simulink model "SEGWAY_RT_SFR"  (R2015a)
settings: Solver=ode4  SolverMode=SingleTasking  StartTime=0.0  StopTime=inf  FixedStep=ts  RelTol=1e-3
values from neighbouring files (symbols this model uses):
  Kcd = place(Ad, Bd, polosd_lc)    [Control_Segway_2015.m]    (also in ensayo1.mat = [-68.2484140277 -10.6212069049 -81.1609824123]; ensayo2_wn4.8_seta_0.7.mat = [-20.5032172519 -3.21085847646 -25.3008871114]; ensayo3_wn5.3_seta_0.55.mat = [-22.2986458352 -3.45646199395 -23.8255259596]; ensayo3_wn5.5_seta_0.7.mat = [-22.2599657852 -3.62971388524 -28.5561648788])
  R = 81.6e-3/2    (= 0.0408)    [CONTROL_SEGWAY.m]    (also in Control_Segway_2015.m; ensayo1.mat; ensayo2_wn4.8_seta_0.7.mat; ensayo3_wn5.3_seta_0.55.mat)
  sound_freq = 440    [CONTROL_SEGWAY.m]    (also in Control_Segway_2015.m; ensayo1.mat; ensayo2_wn4.8_seta_0.7.mat; ensayo3_wn5.3_seta_0.55.mat)
  time_start = 1    [CONTROL_SEGWAY.m]    (also in Control_Segway_2015.m; ensayo1.mat; ensayo2_wn4.8_seta_0.7.mat; ensayo3_wn5.3_seta_0.55.mat)
  ts = 5e-3    (= 0.005)    [CONTROL_SEGWAY.m]    (also in Control_Segway_2015.m; ensayo1.mat; ensayo2_wn4.8_seta_0.7.mat; ensayo3_wn5.3_seta_0.55.mat)
  W = 0.15    [CONTROL_SEGWAY.m]    (also in Control_Segway_2015.m; ensayo1.mat; ensayo2_wn4.8_seta_0.7.mat; ensayo3_wn5.3_seta_0.55.mat)
undefined symbols (not defined in the file or in its folder): th
undefined symbols (not defined in the file): alfa1, gyro0
libraries: legonxtlib x16, simulink x4
settings Model: SimulationMode=external  CovSFcnEnable=off  ExtModeTrigDuration=2  Creator=jrperez  LastModifiedBy=stic
settings DataIOCC: SignalLoggingSaveFormat=ModelDataLogs
settings OptimizationCC: ExpressionDepthLimit=2147483647  OptimizeModelRefInitCode=on  LifeSpan=1
settings DebuggingCC: UnderspecifiedInitializationDetection=Classic  MergeDetectMultiDrivingBlocksExec=none  ParameterPrecisionLossMsg=none  FcnCallInpInsideContextMsg=EnableAllAsWarning  StateNameClashWarn=warning
settings HardwareCC: ProdLargestAtomicInteger=Long  ProdLargestAtomicFloat=Float  ProdEndianess=LittleEndian  ProdHWDeviceType=ARM Compatible->ARM 7
settings RTWCC: SystemTargetFile=realtime.tlc  GenerateMakefile=off  TemplateMakefile=realtime.tmf  Description=Real-Time Toolbox  RTWVerbose=off
settings CodeAppCC: CustomSymbolStrType=$N$R$M  InternalIdentifier=Classic
settings ERTTargetCC: CombineOutputUpdateFcns=off  ExtMode=on  ExtModeTransport=1  ExtModeMexFile=ext_serial_win32_comm_no_acks_rtt_byteswap  ExtModeMexArgs=0 4 9600  ERTSrcFileBannerTemplate=realtime_code_template.cgt  ERTHdrFileBannerTemplate=realtime_code_template.cgt  ERTDataSrcFileTemplate=realtime_code_template.cgt  ERTDataHdrFileTemplate=realtime_code_template.cgt  ERTCustomFileTemplate=realtime_file_process.tlc

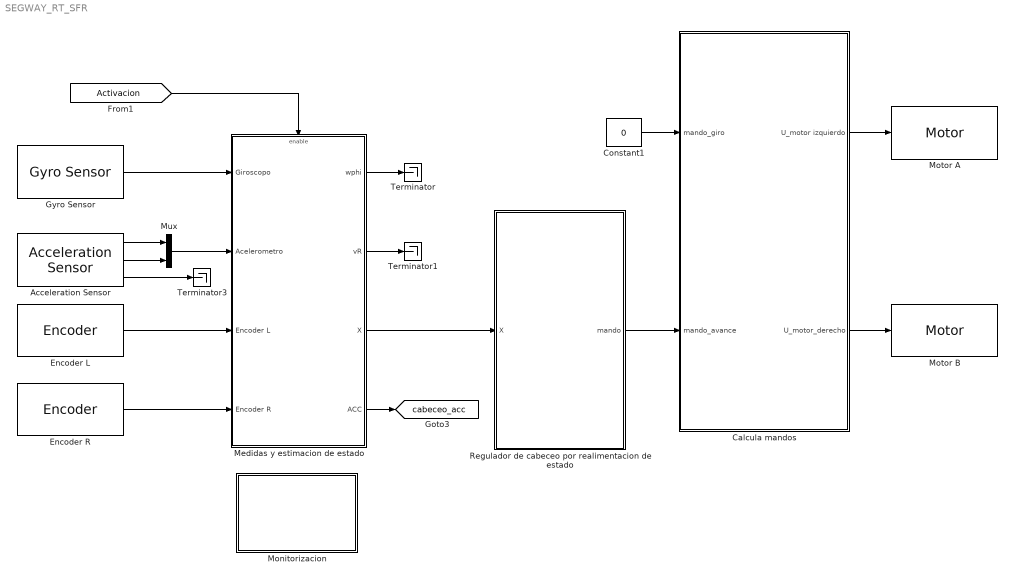
== system SEGWAY_RT_SFR ==
  Acceleration Sensor : legonxtlib/Acceleration Sensor  portNumber=2  sampleTime=ts  blockPlatform=LegoMindstormsNXT
  Calcula mandos : Subsystem
  Constant1 : Constant  Value=0  OutDataTypeStr=single  SampleTime=ts
  Encoder L : legonxtlib/Encoder  portNumber=B  opMode=No reset  sampleTime=ts  blockPlatform=LegoMindstormsNXT
  Encoder R : legonxtlib/Encoder  portNumber=C  opMode=No reset  sampleTime=ts  blockPlatform=LegoMindstormsNXT
  Gyro Sensor : legonxtlib/Gyro Sensor  portNumber=3  outputMode=Raw A/D (0 - 1023)  offset=600  sampleTime=ts  blockPlatform=LegoMindstormsNXT
  Medidas y estimacion de estado : Subsystem
  Monitorizacion : Subsystem
  Motor A : legonxtlib/Motor  sportNumber=B  sstopAction=Brake  blockPlatform=LegoMindstormsNXT
  Motor B : legonxtlib/Motor  sportNumber=C  sstopAction=Brake  blockPlatform=LegoMindstormsNXT
  Mux : Mux  Inputs=2
  Regulador de cabeceo por realimentacion de estado : Subsystem
  Terminator : Terminator
  Terminator1 : Terminator
  Terminator3 : Terminator
  tag scope: cabeceo_acc=global
  wires:
  Gyro Sensor/1 -> Medidas y estimacion de estado/1(Giroscopo)
  Encoder L/1 -> Medidas y estimacion de estado/3(Encoder L)
  Calcula mandos/1(U_motor izquierdo) -> Motor A/1
  Calcula mandos/2(U_motor_derecho) -> Motor B/1
  Encoder R/1 -> Medidas y estimacion de estado/4(Encoder R)
  Medidas y estimacion de estado/3(X) -> Regulador de cabeceo por realimentacion de estado/1(X)
  [Activacion] -> Medidas y estimacion de estado/Enable
  Constant1/1 -> Calcula mandos/1(mando_giro)
  Regulador de cabeceo por realimentacion de estado/1(mando) -> Calcula mandos/2(mando_avance)
  Medidas y estimacion de estado/1(wphi) -> Terminator/1
  Medidas y estimacion de estado/2(vR) -> Terminator1/1
  Acceleration Sensor/3 -> Terminator3/1
  Medidas y estimacion de estado/4(ACC) -> [cabeceo_acc]
  Acceleration Sensor/1 -> Mux/1
  Acceleration Sensor/2 -> Mux/2
  Mux/1 -> Medidas y estimacion de estado/2(Acelerometro)

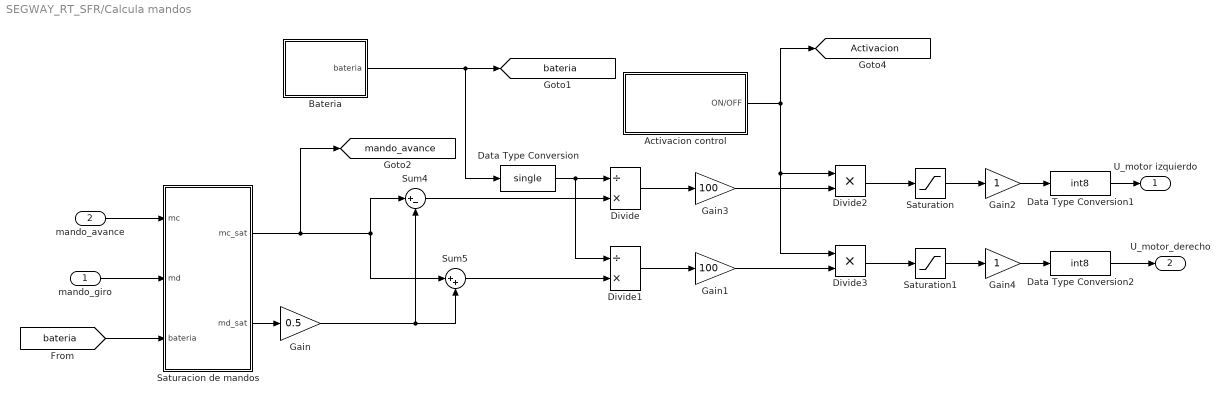
== system SEGWAY_RT_SFR/Calcula mandos ==
  mando_giro : Inport
  mando_avance : Inport  Port=2
  Activacion control : Subsystem
  Bateria : Subsystem
  Data Type Conversion : DataTypeConversion  OutDataTypeStr=single  SampleTime=ts
  Data Type Conversion1 : DataTypeConversion  OutDataTypeStr=int8
  Data Type Conversion2 : DataTypeConversion  OutDataTypeStr=int8
  Divide : Product  Inputs=/*  SampleTime=ts
  Divide1 : Product  Inputs=/*  SampleTime=ts
  Divide2 : Product  SampleTime=ts
  Divide3 : Product  SampleTime=ts
  Gain : Gain  Gain=0.5  OutDataTypeStr=single
  Gain1 : Gain  Gain=100
  Gain2 : Gain
  Gain3 : Gain  Gain=100
  Gain4 : Gain
  Saturacion de mandos : Subsystem
  Saturation : Saturate  UpperLimit=100  LowerLimit=-100
  Saturation1 : Saturate  UpperLimit=100  LowerLimit=-100
  Sum4 : Sum  Inputs=|+-
  Sum5 : Sum  Inputs=|++
  U_motor izquierdo : Outport
  U_motor_derecho : Outport  Port=2
  tag scope: Activacion=global, bateria=global, mando_avance=global
  wires:
  Divide/1 -> Gain3/1
  Sum4/1 -> Divide/2
  Gain3/1 -> Divide2/2
  Divide1/1 -> Gain1/1
  Sum5/1 -> Divide1/2
  Saturacion de mandos/1(mc_sat) -> Sum4/1, Sum5/1, [mando_avance]
  Saturacion de mandos/2(md_sat) -> Gain/1
  Bateria/1(bateria) -> Data Type Conversion/1, [bateria]
  Divide2/1 -> Saturation/1
  Divide3/1 -> Saturation1/1
  Data Type Conversion1/1 -> U_motor izquierdo/1
  Data Type Conversion2/1 -> U_motor_derecho/1
  Data Type Conversion/1 -> Divide/1, Divide1/1
  Gain1/1 -> Divide3/2
  Saturation/1 -> Gain2/1
  Saturation1/1 -> Gain4/1
  [bateria] -> Saturacion de mandos/3(bateria)
  mando_avance/1 -> Saturacion de mandos/1(mc)
  mando_giro/1 -> Saturacion de mandos/2(md)
  Activacion control/1(ON/OFF) -> [Activacion], Divide2/1, Divide3/1
  Gain/1 -> Sum4/2, Sum5/2
  Gain2/1 -> Data Type Conversion1/1
  Gain4/1 -> Data Type Conversion2/1

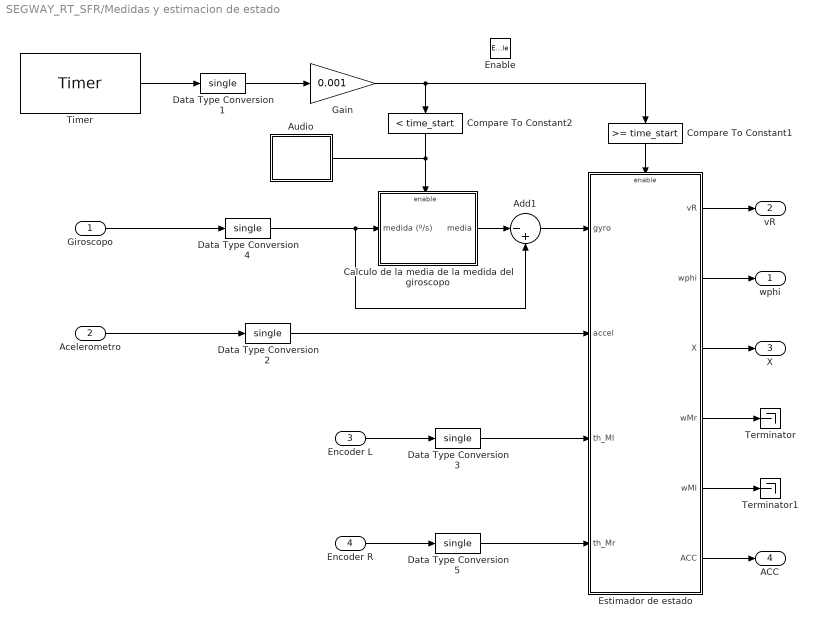
== system SEGWAY_RT_SFR/Medidas y estimacion de estado ==
  Giroscopo : Inport
  Acelerometro : Inport  Port=2
  Encoder L : Inport  Port=3
  Encoder R : Inport  Port=4
  Enable : EnablePort
  Add1 : Sum  Inputs=|-+
  Audio : Subsystem
  Calculo de la media de la medida del giroscopo : Subsystem
  Compare To Constant1 : simulink/Logic and Bit Operations/Compare To Constant  relop=>=  const=time_start  OutDataTypeStr=boolean
  Compare To Constant2 : simulink/Logic and Bit Operations/Compare To Constant  relop=<  const=time_start  OutDataTypeStr=boolean
  Data Type Conversion{1..5} (5 alike) : DataTypeConversion  OutDataTypeStr=single  RndMeth=Simplest
      settings: AttributesFormatString=Round = %<RndMeth>
  Estimador de estado : Subsystem
  Gain : Gain  Gain=0.001
  Terminator : Terminator
  Terminator1 : Terminator
  Timer : legonxtlib/Timer  sampleTime=ts  blockPlatform=LegoMindstormsNXT
  wphi : Outport
  vR : Outport  Port=2
  X : Outport  Port=3
  ACC : Outport  Port=4
  wires:
  Data Type Conversion4/1 -> Calculo de la media de la medida del giroscopo/1(medida (º/s)), Add1/2
  Calculo de la media de la medida del giroscopo/1(media) -> Add1/1
  Giroscopo/1 -> Data Type Conversion4/1
  Compare To Constant2/1 -> Calculo de la media de la medida del giroscopo/Enable, Audio/Enable
  Encoder L/1 -> Data Type Conversion3/1
  Encoder R/1 -> Data Type Conversion5/1
  Add1/1 -> Estimador de estado/1(gyro)
  Data Type Conversion3/1 -> Estimador de estado/3(th_Ml)
  Data Type Conversion5/1 -> Estimador de estado/4(th_Mr)
  Estimador de estado/5(wMl) -> Terminator1/1
  Estimador de estado/4(wMr) -> Terminator/1
  Estimador de estado/1(vR) -> vR/1
  Estimador de estado/2(wphi) -> wphi/1
  Estimador de estado/3(X) -> X/1
  Gain/1 -> Compare To Constant2/1, Compare To Constant1/1
  Timer/1 -> Data Type Conversion1/1
  Compare To Constant1/1 -> Estimador de estado/Enable
  Data Type Conversion1/1 -> Gain/1
  Data Type Conversion2/1 -> Estimador de estado/2(accel)
  Acelerometro/1 -> Data Type Conversion2/1
  Estimador de estado/6(ACC) -> ACC/1

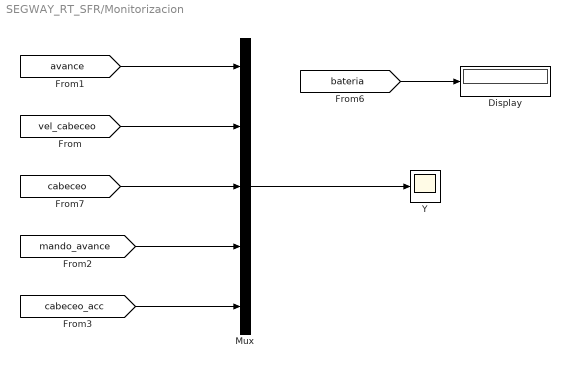
== system SEGWAY_RT_SFR/Monitorizacion ==
  Display : Display
  Mux : Mux  Inputs=5
  Y : Scope
      settings: TimeRange=10  YMin=-3.5  YMax=7.5  SaveName=Y  SampleTime=0.1
  wires:
  [bateria] -> Display/1
  Mux/1 -> Y/1
  [cabeceo] -> Mux/3
  [mando_avance] -> Mux/4
  [vel_cabeceo] -> Mux/2
  [avance] -> Mux/1
  [cabeceo_acc] -> Mux/5

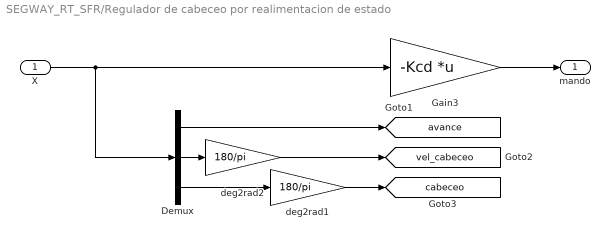
== system SEGWAY_RT_SFR/Regulador de cabeceo por realimentacion de estado ==
  X : Inport  SampleTime=ts
  Demux : Demux  Outputs=3
  Gain3 : Gain  Gain=-Kcd  Multiplication=Matrix(K*u) (u vector)  SaturateOnIntegerOverflow=on  OutDataTypeStr=Inherit: Same as input  ParamDataTypeStr=Inherit: Same as input
  deg2rad1 : Gain  Gain=180/pi  OutDataTypeStr=Inherit: Same as input  ParamDataTypeStr=Inherit: Same as input
  deg2rad2 : Gain  Gain=180/pi  OutDataTypeStr=Inherit: Same as input  ParamDataTypeStr=Inherit: Same as input
  mando : Outport
  tag scope: avance=global, cabeceo=global, vel_cabeceo=global
  wires:
  Gain3/1 -> mando/1
  X/1 -> Gain3/1, Demux/1
  Demux/1 -> [avance]
  Demux/2 -> deg2rad2/1
  Demux/3 -> deg2rad1/1
  deg2rad1/1 -> [cabeceo]
  deg2rad2/1 -> [vel_cabeceo]

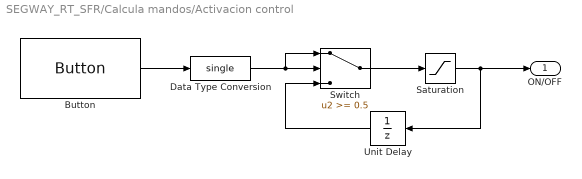
== system SEGWAY_RT_SFR/Calcula mandos/Activacion control ==
  Button : legonxtlib/Button  buttonType=Middle orange  sampleTime=0.1  blockPlatform=LegoMindstormsNXT
  Data Type Conversion : DataTypeConversion  OutDataTypeStr=single
  Saturation : Saturate  UpperLimit=1  LowerLimit=0
  Switch : Switch  Threshold=0.5
  Unit Delay : UnitDelay  SampleTime=0.1
  ON/OFF : Outport
  wires:
  Button/1 -> Data Type Conversion/1
  Switch/1 -> Saturation/1
  Unit Delay/1 -> Switch/3
  Data Type Conversion/1 -> Switch/2, Switch/1
  Saturation/1 -> Unit Delay/1, ON/OFF/1

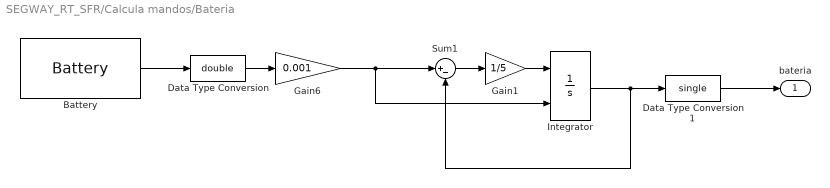
== system SEGWAY_RT_SFR/Calcula mandos/Bateria ==
  Battery : legonxtlib/Battery  sampleTime=0.1  blockPlatform=LegoMindstormsNXT
  Data Type Conversion : DataTypeConversion  OutDataTypeStr=double
  Data Type Conversion1 : DataTypeConversion  OutDataTypeStr=single
  Gain1 : Gain  Gain=1/5
  Gain6 : Gain  Gain=0.001
  Integrator : Integrator  InitialConditionSource=external
  Sum1 : Sum  Inputs=|+-
  bateria : Outport
  wires:
  Battery/1 -> Data Type Conversion/1
  Data Type Conversion/1 -> Gain6/1
  Sum1/1 -> Gain1/1
  Integrator/1 -> Sum1/2, Data Type Conversion1/1
  Gain6/1 -> Sum1/1, Integrator/2
  Gain1/1 -> Integrator/1
  Data Type Conversion1/1 -> bateria/1

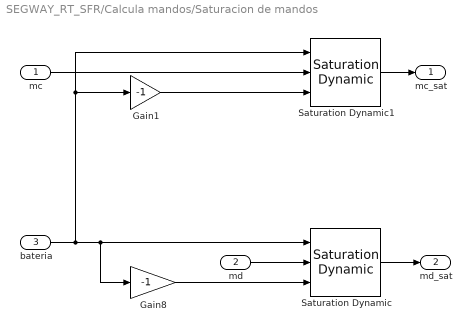
== system SEGWAY_RT_SFR/Calcula mandos/Saturacion de mandos ==
  mc : Inport
  md : Inport  Port=2
  bateria : Inport  Port=3  SampleTime=ts
  Gain1 : Gain  Gain=-1
  Gain8 : Gain  Gain=-1
  Saturation Dynamic : simulink/Discontinuities/Saturation Dynamic  OutMin=[]  OutMax=[]  OutDataTypeStr=Inherit: Same as second input  OutDataType=fixdt(1, 16)  OutScaling=2^-10  DoSatur=off
  Saturation Dynamic1 : simulink/Discontinuities/Saturation Dynamic  OutMin=[]  OutMax=[]  OutDataTypeStr=Inherit: Same as second input  OutDataType=fixdt(1, 16)  OutScaling=2^-10  DoSatur=off
  mc_sat : Outport
  md_sat : Outport  Port=2
  wires:
  Saturation Dynamic1/1 -> mc_sat/1
  Gain8/1 -> Saturation Dynamic/3
  mc/1 -> Saturation Dynamic1/2
  md/1 -> Saturation Dynamic/2
  Saturation Dynamic/1 -> md_sat/1
  bateria/1 -> Gain1/1, Saturation Dynamic1/1, Gain8/1, Saturation Dynamic/1
  Gain1/1 -> Saturation Dynamic1/3

== system SEGWAY_RT_SFR/Medidas y estimacion de estado/Audio ==
  Enable : EnablePort
  Constant2 : Constant  Value=sound_freq  OutDataTypeStr=single  SampleTime=0.2
      settings: AttributesFormatString=DataType = %<OutDataTypeStr>
  Speaker : legonxtlib/Speaker  sinputMode=Frequency only  sspeakerFreq=100  sspeakerVolume=50  sspeakerDuration=100  blockPlatform=LegoMindstormsNXT
  wires:
  Constant2/1 -> Speaker/1

== system SEGWAY_RT_SFR/Medidas y estimacion de estado/Calculo de la media de la medida del giroscopo ==
  medida (º/s) : Inport  SampleTime=ts
  Enable : EnablePort
  Filtro digital paso bajo : Subsystem  mask{alfa=alfa1, x0=gyro0, ts=ts}
      mask prompts: alfa "Constante de filtrado"; x0 "Condición inicial"; ts "Período de muestreo"
  media : Outport
  wires:
  medida (º/s)/1 -> Filtro digital paso bajo/1(ent)
  Filtro digital paso bajo/1(sal) -> media/1

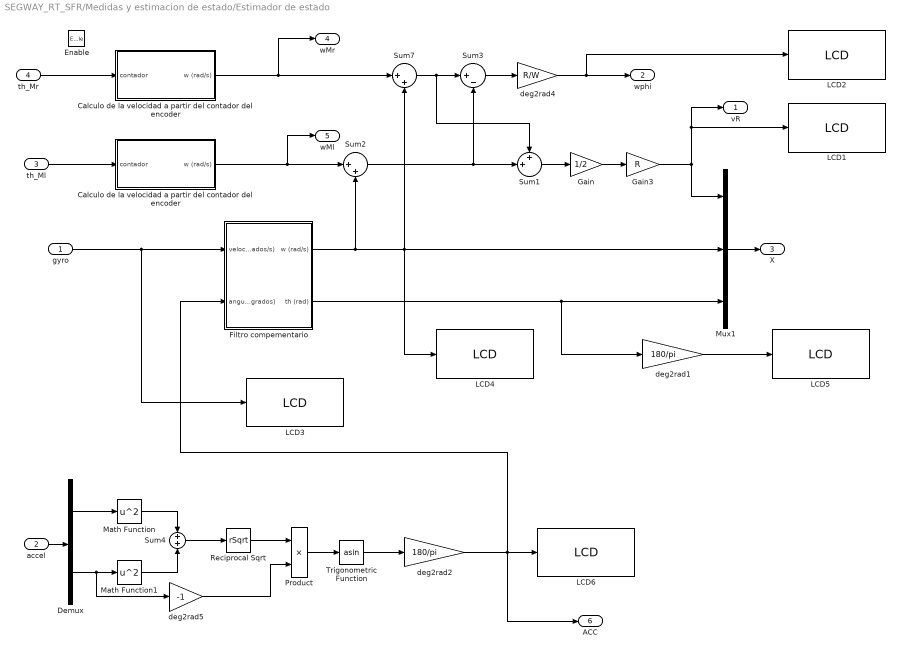
== system SEGWAY_RT_SFR/Medidas y estimacion de estado/Estimador de estado ==
  gyro : Inport
  accel : Inport  Port=2
  th_Ml : Inport  Port=3
  th_Mr : Inport  Port=4
  Enable : EnablePort
  Calculo de la velocidad a partir del contador del encoder : Subsystem  mask{GpT=1, alfa=alfa1, ts=ts}
      mask prompts: GpT "grados/tick"; alfa "Constante de filtrado paso bajo"; ts "Período de muestreo"
  "Calculo de la velocidad a partir del contador del encoder " : Subsystem  mask{GpT=1, alfa=alfa1, ts=ts}
      mask prompts: GpT "grados/tick"; alfa "Constante de filtrado paso bajo"; ts "Período de muestreo"
  Demux : Demux  Outputs=2
  Filtro compementario : Subsystem
  Gain : Gain  Gain=1/2  OutDataTypeStr=Inherit: Same as input  ParamDataTypeStr=Inherit: Same as input
  Gain3 : Gain  Gain=R  OutDataTypeStr=Inherit: Same as input  ParamDataTypeStr=Inherit: Same as input
  LCD1 : legonxtlib/LCD  slcdStr=vR  slcdLine=1  slcdFormat=Decimal  blockPlatform=LegoMindstormsNXT
  LCD2 : legonxtlib/LCD  slcdStr=wphi  slcdLine=2  slcdFormat=Decimal  blockPlatform=LegoMindstormsNXT
  LCD3 : legonxtlib/LCD  slcdStr=gyro  slcdLine=3  slcdFormat=Decimal  blockPlatform=LegoMindstormsNXT
  LCD4 : legonxtlib/LCD  slcdStr=wth  slcdLine=4  slcdFormat=Decimal  blockPlatform=LegoMindstormsNXT
  LCD5 : legonxtlib/LCD  slcdStr=th (º)  slcdLine=5  slcdFormat=Decimal  blockPlatform=LegoMindstormsNXT
  LCD6 : legonxtlib/LCD  slcdStr=tha  slcdLine=6  slcdFormat=Decimal  blockPlatform=LegoMindstormsNXT
  Math Function : Math  Operator=square  SaturateOnIntegerOverflow=on
  Math Function1 : Math  Operator=square  SaturateOnIntegerOverflow=on
  Mux1 : Mux  Inputs=3
  Product : Product
  Reciprocal Sqrt : Sqrt  Operator=rSqrt  SaturateOnIntegerOverflow=on
  Sum1 : Sum  Inputs=++|  OutDataTypeStr=Inherit: Same as first input
  Sum2 : Sum  Inputs=|++  OutDataTypeStr=Inherit: Same as first input
  Sum3 : Sum  Inputs=|+-
  Sum4 : Sum  Inputs=+|+
  Sum7 : Sum  Inputs=|++
  Trigonometric Function : Trigonometry  Operator=asin
  deg2rad1 : Gain  Gain=180/pi  OutDataTypeStr=Inherit: Same as input  ParamDataTypeStr=Inherit: Same as input
  deg2rad2 : Gain  Gain=180/pi  OutDataTypeStr=Inherit: Same as input  ParamDataTypeStr=Inherit: Same as input
  deg2rad4 : Gain  Gain=R/W  OutDataTypeStr=Inherit: Same as input  ParamDataTypeStr=Inherit: Same as input
  deg2rad5 : Gain  Gain=-1  OutDataTypeStr=Inherit: Same as input  ParamDataTypeStr=Inherit: Same as input
  vR : Outport
  wphi : Outport  Port=2
  X : Outport  Port=3
  wMr : Outport  Port=4
  wMl : Outport  Port=5
  ACC : Outport  Port=6
  wires:
  gyro/1 -> LCD3/1, Filtro compementario/1(velocidad (grados/s))
  Sum2/1 -> Sum1/2, Sum3/2
  Sum7/1 -> Sum1/1, Sum3/1
  Sum3/1 -> deg2rad4/1
  Calculo de la velocidad a partir del contador del encoder/1(w (rad/s)) -> Sum2/1, wMl/1
  "Calculo de la velocidad a partir del contador del encoder "/1(w (rad/s)) -> Sum7/1, wMr/1
  Sum1/1 -> Gain/1
  Mux1/1 -> X/1
  th_Ml/1 -> Calculo de la velocidad a partir del contador del encoder/1(contador)
  th_Mr/1 -> "Calculo de la velocidad a partir del contador del encoder "/1(contador)
  deg2rad4/1 -> wphi/1, LCD2/1
  Gain3/1 -> Mux1/1, LCD1/1, vR/1
  Gain/1 -> Gain3/1
  Filtro compementario/1(w (rad/s)) -> Sum7/2, Mux1/2, LCD4/1, Sum2/2
  Filtro compementario/2(th (rad)) -> Mux1/3, deg2rad1/1
  deg2rad1/1 -> LCD5/1
  Trigonometric Function/1 -> deg2rad2/1
  deg2rad2/1 -> ACC/1, Filtro compementario/2(angulo (grados)), LCD6/1
  accel/1 -> Demux/1
  Demux/1 -> Math Function/1
  Math Function/1 -> Sum4/1
  Math Function1/1 -> Sum4/2
  Sum4/1 -> Reciprocal Sqrt/1
  Reciprocal Sqrt/1 -> Product/1
  Demux/2 -> deg2rad5/1, Math Function1/1
  deg2rad5/1 -> Product/2
  Product/1 -> Trigonometric Function/1

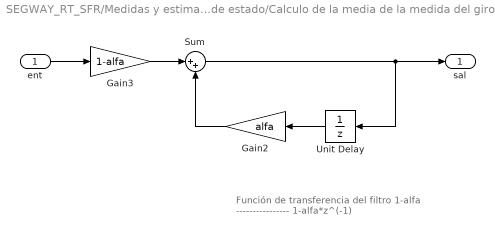
== system SEGWAY_RT_SFR/Medidas y estimacion de estado/Calculo de la media de la medida del giroscopo/Filtro digital paso bajo ==
  note: Función de transferencia del filtro
      |                        1-alfa
      |                  ----------------
      |                   1-alfa*z^(-1)
  ent : Inport  SampleTime=ts
  Gain2 : Gain  Gain=alfa  OutDataTypeStr=Inherit: Same as input  ParamDataTypeStr=Inherit: Same as input
  Gain3 : Gain  Gain=1-alfa  OutDataTypeStr=Inherit: Same as input  ParamDataTypeStr=Inherit: Same as input
  Sum : Sum  Inputs=|++  OutDataTypeStr=Inherit: Same as first input
  Unit Delay : UnitDelay  InitialCondition=x0  SampleTime=-1
  sal : Outport
  wires:
  ent/1 -> Gain3/1
  Gain3/1 -> Sum/1
  Gain2/1 -> Sum/2
  Unit Delay/1 -> Gain2/1
  Sum/1 -> sal/1, Unit Delay/1

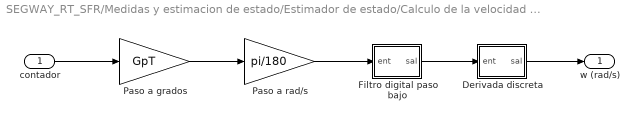
== system SEGWAY_RT_SFR/Medidas y estimacion de estado/Estimador de estado/Calculo de la velocidad a partir del contador del encoder ==
  contador : Inport  SampleTime=ts
  Derivada discreta : Subsystem  mask{ts=ts, opcion=Derivada en adelanto s=(1-z^-1)/ts}
      mask prompts: ts "Período de muestreo"; opcion "Método de discretización"
      mask init:
      | z=tf('z',ts);
      | switch(opcion)
      |     case 1
      |         derivada=minreal((1-z^-1)/ts);
      |     case 2
      |         derivada=minreal(2*(1-z^-1)/ts/(1+z^-1));
      |     case 3
      |         derivada=minreal((1.5-2*z^-1+0.5*z^-2)/ts);
      | end
      mask TypeOptions opcion: Derivada en adelanto s=(1-z^-1)/ts  | Trapezoidal s=2*(1-z^-1)/ts/(1+z^-1) | Derivada por aproximación parabólica s=(1.5-2*z^-1+0.5z^-2)/ts
  Filtro digital paso bajo : Subsystem  mask{alfa=alfa, x0=0, ts=ts}
      mask prompts: alfa "Constante de filtrado"; x0 "Condición inicial"; ts "Período de muestreo"
  Paso a grados : Gain  Gain=GpT
  Paso a rad/s : Gain  Gain=pi/180
  w (rad/s) : Outport
  wires:
  contador/1 -> Paso a grados/1
  Paso a grados/1 -> Paso a rad/s/1
  Paso a rad/s/1 -> Filtro digital paso bajo/1(ent)
  Filtro digital paso bajo/1(sal) -> Derivada discreta/1(ent)
  Derivada discreta/1(sal) -> w (rad/s)/1

== system SEGWAY_RT_SFR/Medidas y estimacion de estado/Estimador de estado/Calculo de la velocidad a partir del contador del encoder  ==
  contador : Inport  SampleTime=ts
  Derivada discreta : Subsystem  mask{ts=ts, opcion=Derivada en adelanto s=(1-z^-1)/ts}
      mask prompts: ts "Período de muestreo"; opcion "Método de discretización"
      mask init: same as SEGWAY_RT_SFR/Medidas y estimacion de estado/Estimador de estado/Calculo de la velocidad a partir del contador del encoder/Derivada discreta
      mask TypeOptions opcion: Derivada en adelanto s=(1-z^-1)/ts  | Trapezoidal s=2*(1-z^-1)/ts/(1+z^-1) | Derivada por aproximación parabólica s=(1.5-2*z^-1+0.5z^-2)/ts
  Filtro digital paso bajo : Subsystem  mask{alfa=alfa, x0=0, ts=ts}
      mask prompts: alfa "Constante de filtrado"; x0 "Condición inicial"; ts "Período de muestreo"
  Paso a grados : Gain  Gain=GpT
  Paso a rad/s : Gain  Gain=pi/180
  w (rad/s) : Outport
  wires:
  Derivada discreta/1(sal) -> w (rad/s)/1
  Filtro digital paso bajo/1(sal) -> Derivada discreta/1(ent)
  Paso a rad/s/1 -> Filtro digital paso bajo/1(ent)
  Paso a grados/1 -> Paso a rad/s/1
  contador/1 -> Paso a grados/1

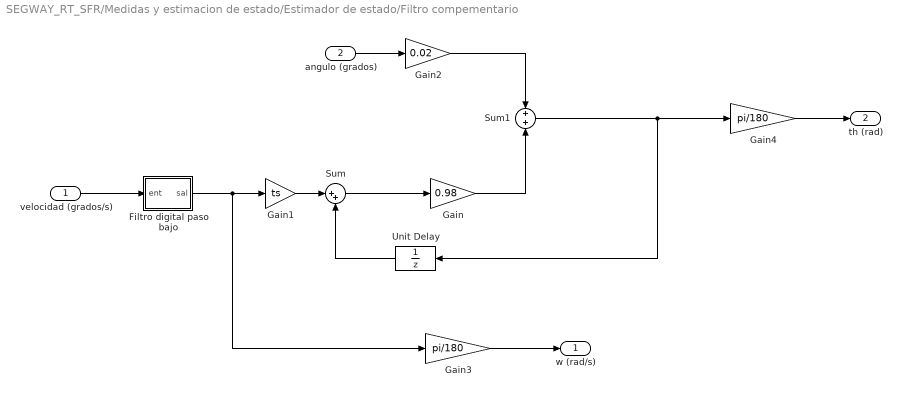
== system SEGWAY_RT_SFR/Medidas y estimacion de estado/Estimador de estado/Filtro compementario ==
  velocidad (grados/s) : Inport  SampleTime=ts
  angulo (grados) : Inport  Port=2  SampleTime=ts
  Filtro digital paso bajo : Subsystem  mask{alfa=alfa1, x0=0, ts=ts}
      mask prompts: alfa "Constante de filtrado"; x0 "Condición inicial"; ts "Período de muestreo"
  Gain : Gain  Gain=0.98
  Gain1 : Gain  Gain=ts
  Gain2 : Gain  Gain=0.02
  Gain3 : Gain  Gain=pi/180
  Gain4 : Gain  Gain=pi/180
  Sum : Sum  Inputs=|++
  Sum1 : Sum  Inputs=+|+
  Unit Delay : UnitDelay  SampleTime=-1
  w (rad/s) : Outport
  th (rad) : Outport  Port=2
  wires:
  Gain1/1 -> Sum/1
  Unit Delay/1 -> Sum/2
  Sum/1 -> Gain/1
  Gain/1 -> Sum1/2
  angulo (grados)/1 -> Gain2/1
  Gain2/1 -> Sum1/1
  Sum1/1 -> Gain4/1, Unit Delay/1
  Gain3/1 -> w (rad/s)/1
  Gain4/1 -> th (rad)/1
  velocidad (grados/s)/1 -> Filtro digital paso bajo/1(ent)
  Filtro digital paso bajo/1(sal) -> Gain3/1, Gain1/1

== system SEGWAY_RT_SFR/Medidas y estimacion de estado/Estimador de estado/Calculo de la velocidad a partir del contador del encoder/Derivada discreta ==
  ent : Inport  SampleTime=ts
  Discrete Transfer Fcn : DiscreteTransferFcn  Numerator=derivada.num{1}  Denominator=derivada.den{1}
  sal : Outport
  wires:
  ent/1 -> Discrete Transfer Fcn/1
  Discrete Transfer Fcn/1 -> sal/1

== system SEGWAY_RT_SFR/Medidas y estimacion de estado/Estimador de estado/Calculo de la velocidad a partir del contador del encoder/Filtro digital paso bajo ==
  note: Función de transferencia del filtro
      |                        1-alfa
      |                  ----------------
      |                   1-alfa*z^(-1)
  ent : Inport  SampleTime=ts
  Gain2 : Gain  Gain=alfa  OutDataTypeStr=Inherit: Same as input  ParamDataTypeStr=Inherit: Same as input
  Gain3 : Gain  Gain=1-alfa  OutDataTypeStr=Inherit: Same as input  ParamDataTypeStr=Inherit: Same as input
  Sum : Sum  Inputs=|++  OutDataTypeStr=Inherit: Same as first input
  Unit Delay : UnitDelay  SampleTime=-1
  sal : Outport
  wires:
  ent/1 -> Gain3/1
  Gain3/1 -> Sum/1
  Gain2/1 -> Sum/2
  Unit Delay/1 -> Gain2/1
  Sum/1 -> sal/1, Unit Delay/1

== system SEGWAY_RT_SFR/Medidas y estimacion de estado/Estimador de estado/Calculo de la velocidad a partir del contador del encoder /Derivada discreta ==
  ent : Inport  SampleTime=ts
  Discrete Transfer Fcn : DiscreteTransferFcn  Numerator=derivada.num{1}  Denominator=derivada.den{1}
  sal : Outport
  wires:
  Discrete Transfer Fcn/1 -> sal/1
  ent/1 -> Discrete Transfer Fcn/1

== system SEGWAY_RT_SFR/Medidas y estimacion de estado/Estimador de estado/Calculo de la velocidad a partir del contador del encoder /Filtro digital paso bajo ==
  note: Función de transferencia del filtro
      |                        1-alfa
      |                  ----------------
      |                   1-alfa*z^(-1)
  ent : Inport  SampleTime=ts
  Gain2 : Gain  Gain=alfa  OutDataTypeStr=Inherit: Same as input  ParamDataTypeStr=Inherit: Same as input
  Gain3 : Gain  Gain=1-alfa  OutDataTypeStr=Inherit: Same as input  ParamDataTypeStr=Inherit: Same as input
  Sum : Sum  Inputs=|++  OutDataTypeStr=Inherit: Same as first input
  Unit Delay : UnitDelay  SampleTime=-1
  sal : Outport
  wires:
  Sum/1 -> Unit Delay/1, sal/1
  Unit Delay/1 -> Gain2/1
  Gain2/1 -> Sum/2
  Gain3/1 -> Sum/1
  ent/1 -> Gain3/1

== system SEGWAY_RT_SFR/Medidas y estimacion de estado/Estimador de estado/Filtro compementario/Filtro digital paso bajo ==
  note: Función de transferencia del filtro
      |                        1-alfa
      |                  ----------------
      |                   1-alfa*z^(-1)
  ent : Inport  SampleTime=ts
  Gain2 : Gain  Gain=alfa  OutDataTypeStr=Inherit: Same as input  ParamDataTypeStr=Inherit: Same as input
  Gain3 : Gain  Gain=1-alfa  OutDataTypeStr=Inherit: Same as input  ParamDataTypeStr=Inherit: Same as input
  Sum : Sum  Inputs=|++  OutDataTypeStr=Inherit: Same as first input
  Unit Delay : UnitDelay  SampleTime=-1
  sal : Outport
  wires:
  Sum/1 -> Unit Delay/1, sal/1
  Unit Delay/1 -> Gain2/1
  Gain2/1 -> Sum/2
  Gain3/1 -> Sum/1
  ent/1 -> Gain3/1
